simulink model "FlightModel"  (R2014a)
settings: Solver=ode45  StartTime=0.0  StopTime=20  RelTol=1e-3
PreLoadFcn:
  | initalize
model workspace: external: MAT-File (data not in the file)
values from neighbouring files (symbols this model uses):
  deltaMass = mass - mass(1)    [generateMotorData.m]
  dt_data = time(2)-time(1)    [generateMotorData.m]
  m0 = 7.6370    (= 7.637)    [generateMotorData.m]    (also in initalize.m)
  thrust = interp1(timeTmp,thrustTmp,time,'spline')    [generateMotorData.m]
libraries: aerolibatmos2 x1
settings Model: Creator=Jack  LastModifiedBy=Jack

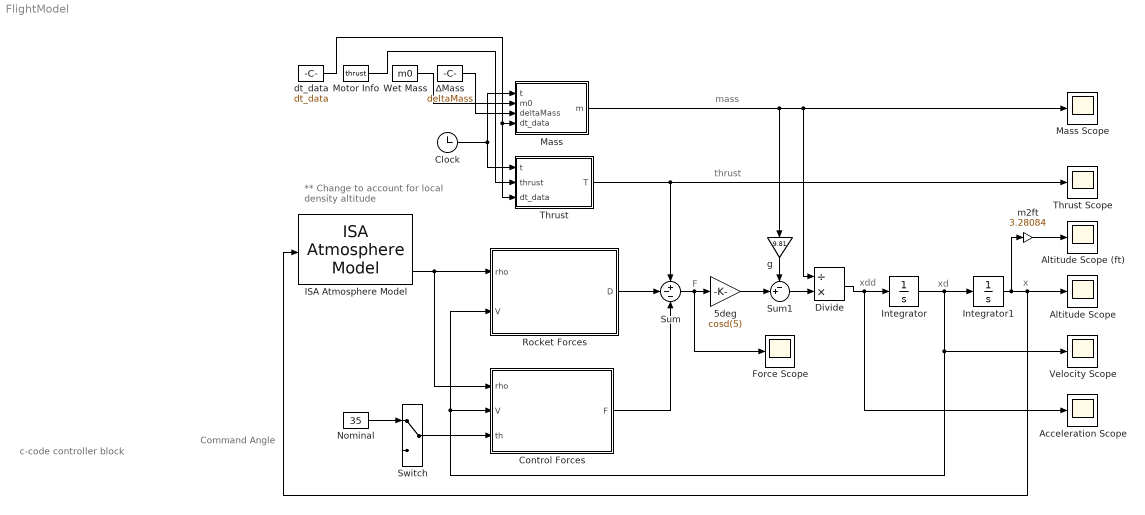
== system FlightModel ==
  note: c-code controller block
  note: mass
  note: ** Change to account
      | for local density altitude
  note: Command Angle
  note: x
  note: xd
  note: xdd
  note: F
  note: thrust
  " Acceleration Scope" : Scope
      settings: SaveName=ScopeData3
  " Altitude Scope" : Scope
  " Altitude Scope (ft)" : Scope
      settings: SaveName=ScopeData6
  " Velocity Scope" : Scope
      settings: SaveName=ScopeData2
  5deg : Gain  Gain=cosd(5)
  Clock : Clock
  Control Forces : MATLAB Function  TreatAsAtomicUnit=on
  Divide : Product  Inputs=/*
  Force Scope : Scope
      settings: SaveName=ScopeData5
  ISA Atmosphere Model : aerolibatmos2/ISA Atmosphere Model  custom=on  g=9.80665  gamma=1.4  R=287.0531  L=0.0065  h_trop=11000  h_strat=20000  rho0=1.225  P0=101325  T0=288.15  h0=0
  Integrator : Integrator
  Integrator1 : Integrator
  Mass : MATLAB Function  TreatAsAtomicUnit=on
  "Mass Scope " : Scope
  Motor Info : Constant  Value=thrust
  Nominal : Constant  Value=35
  Rocket Forces : MATLAB Function  TreatAsAtomicUnit=on
  Sum : Sum  Inputs=+--
  Sum1 : Sum  Inputs=-+|
  Switch : ManualSwitch
  Thrust : MATLAB Function  TreatAsAtomicUnit=on
  Thrust Scope : Scope
      settings: SaveName=ScopeData4
  Wet Mass : Constant  Value=m0
  dt_data : Constant  Value=dt_data
  g : Gain  Gain=9.81
  m2ft : Gain  Gain=3.28084
  ∆Mass : Constant  Value=deltaMass  OutDataTypeStr=Inherit: Inherit via back propagation
  wires:
  ISA Atmosphere Model/4 -> Rocket Forces/1(rho), Control Forces/1(rho)
  Divide/1 -> " Acceleration Scope"/1, Integrator/1
  Integrator/1 -> Integrator1/1, Rocket Forces/2(V), Control Forces/2(V), " Velocity Scope"/1
  Integrator1/1 -> m2ft/1, " Altitude Scope"/1, ISA Atmosphere Model/1
  Switch/1 -> Control Forces/3(th)
  Nominal/1 -> Switch/1
  Clock/1 -> Mass/1(t), Thrust/1(t)
  Thrust/1(T) -> Thrust Scope/1, Sum/1
  Rocket Forces/1(D) -> Sum/2
  Control Forces/1(F) -> Sum/3
  Sum/1 -> Force Scope/1, 5deg/1
  Sum1/1 -> Divide/2
  Mass/1(m) -> "Mass Scope "/1, Divide/1, g/1
  5deg/1 -> Sum1/2
  g/1 -> Sum1/1
  ? -> Switch/2
  Wet Mass/1 -> Mass/2(m0)
  Motor Info/1 -> Thrust/2(thrust)
  dt_data/1 -> Thrust/3(dt_data), Mass/4(dt_data)
  ∆Mass/1 -> Mass/3(deltaMass)
  m2ft/1 -> " Altitude Scope (ft)"/1

== matlab function FlightModel/Control Forces ==
  data: rho input; F output; V input; th input
function F = sumControlForces(rho, V, th)
S = .0007;
% c_d = fn(th)
c_d = 1;
F = .5*rho*V^2*S*c_d;

== matlab function FlightModel/Rocket Forces ==
  data: rho input; D output; V input
%% Sum forces on rocket
function D = sumRocketForces(rho, V)
% c_d = c_d_0 + c_d_alpha * aoa
% c_l = c_l_0 + c_l_alpha * aoa
S = .0082;
c_d = .5;
D = .5*rho*V^2*S*c_d;

== matlab function FlightModel/Thrust ==
  data: t input; T output; thrust input; dt_data input
function T = thrust(t, thrust, dt_data)
% Index loaded thrust array, dt_data loaded with thrust data.
%global thrust dt_data;
ndx = floor(t/dt_data);
if ndx == 0
    ndx = 1;
elseif ndx > length(thrust)
    ndx = length(thrust);
end
T = thrust(ndx);

== matlab function FlightModel/Mass ==
  data: t input; m output; m0 input; deltaMass input; dt_data input
function m = massUpdate(t, m0, deltaMass, dt_data)
% Index loaded mass array, dt_data loaded with mass data.
%global deltaMass dt_data m0;
ndx = floor(t/dt_data);
if ndx == 0
    ndx = 1;
elseif ndx > length(deltaMass)
    ndx = length(deltaMass);
end
m = m0 - deltaMass(ndx);
